simulink model "BallPlate"  (R2018b)
settings: Solver=VariableStepAuto  StartTime=0.0  StopTime=20  FixedStep=0.001  RelTol=1e-3
libraries: vrlib x6, aerolibanimutils x1
settings Model: Creator=enrico  LastModifiedBy=enrico

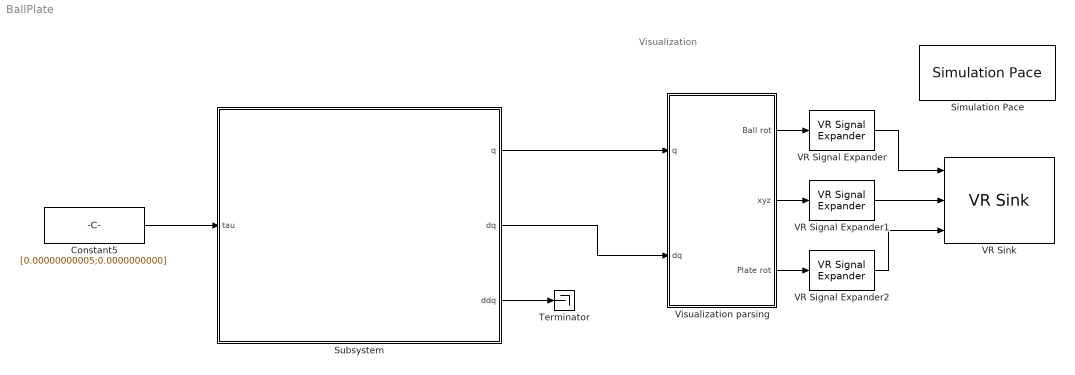
== system BallPlate ==
  note: Visualization
  Constant5 : Constant  Value=[0.00000000005;0.0000000000]
  Simulation Pace : aerolibanimutils/Simulation Pace  SimulationPace=1  SleepMode=Auto  OutputPaceError=off  SampleTime=1/30
  Subsystem : Subsystem
  Terminator : Terminator
  VR Signal Expander : vrlib/VR Signal Expander  outwidth=4  outidx=[1 2 3 4]
      settings: SourceProductName=Simulink 3D Animation  SourceProductBaseCode=VR
  VR Signal Expander1 : vrlib/VR Signal Expander  outwidth=3  outidx=[1 2 3]
      settings: SourceProductName=Simulink 3D Animation  SourceProductBaseCode=VR
  VR Signal Expander2 : vrlib/VR Signal Expander  outwidth=4  outidx=[1 2 3 4]
      settings: SourceProductName=Simulink 3D Animation  SourceProductBaseCode=VR
  VR Sink : vrlib/VR Sink  InstantiateOnLoad=on  SampleTime=-1  ViewEnable=on  RemoteChange=off  RemoteView=off  FieldsWritten=Ball.rotation.4.1.1.double#Ball.translation.3.1.1.double#Plate.rotation.4.1.1.double  WorldFileName=BallPlateVR.wrl  WorldDescription=Ball and plate  AutoView=on  VideoDimensions=[]  AllowVariableSize=off  mask(Virtual Reality Sink){}
      settings: SourceProductBaseCode=VR
  Visualization parsing : Subsystem
  wires:
  VR Signal Expander/1 -> VR Sink/1
  VR Signal Expander2/1 -> VR Sink/3
  Subsystem/1(q) -> Visualization parsing/1(q)
  Subsystem/2(dq) -> Visualization parsing/2(dq)
  Visualization parsing/1(Ball rot) -> VR Signal Expander/1
  VR Signal Expander1/1 -> VR Sink/2
  Subsystem/3(ddq) -> Terminator/1
  Visualization parsing/2(xyz) -> VR Signal Expander1/1
  Visualization parsing/3(Plate rot) -> VR Signal Expander2/1
  Constant5/1 -> Subsystem/1(tau)

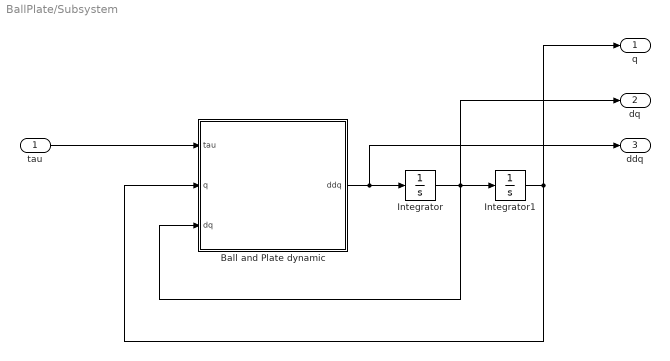
== system BallPlate/Subsystem ==
  tau : Inport
  Ball and Plate dynamic : MATLAB Function  TreatAsAtomicUnit=on
  Integrator : Integrator  InitialCondition=[0; 0; 0; 0]
  Integrator1 : Integrator  InitialCondition=[0; 0; 0; 0]
  q : Outport
  dq : Outport  Port=2
  ddq : Outport  Port=3
  wires:
  tau/1 -> Ball and Plate dynamic/1(tau)
  Integrator1/1 -> q/1, Ball and Plate dynamic/2(q)
  Integrator/1 -> Ball and Plate dynamic/3(dq), dq/1, Integrator1/1
  Ball and Plate dynamic/1(ddq) -> ddq/1, Integrator/1

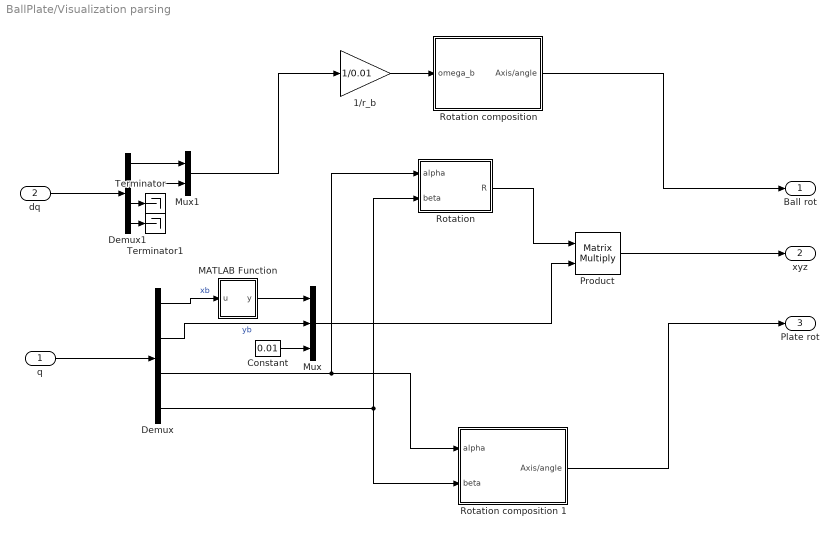
== system BallPlate/Visualization parsing ==
  q : Inport
  dq : Inport  Port=2
  1/r_b : Gain  Gain=1/0.01
  Constant : Constant  Value=0.01
  Demux : Demux
  Demux1 : Demux
  MATLAB Function : MATLAB Function  TreatAsAtomicUnit=on
  Mux : Mux  Inputs=3
  Mux1 : Mux  Inputs=2
  Product : Product  Multiplication=Matrix(*)
  Rotation : MATLAB Function  TreatAsAtomicUnit=on
  Rotation composition : Subsystem
  Rotation composition 1 : Subsystem
  Terminator : Terminator
  Terminator1 : Terminator
  Ball rot : Outport
  xyz : Outport  Port=2
  Plate rot : Outport  Port=3
  wires:
  Demux/2 -> Mux/2  "yb"
  1/r_b/1 -> Rotation composition/1(omega_b)
  Demux/3 -> Rotation/1(alpha), Rotation composition 1/1(alpha)
  dq/1 -> Demux1/1
  Mux1/1 -> 1/r_b/1
  Demux/1 -> MATLAB Function/1(u)  "xb"
  q/1 -> Demux/1
  Demux1/1 -> Mux1/1
  Demux1/4 -> Terminator1/1
  Rotation composition/1(Axis/angle) -> Ball rot/1
  Demux1/3 -> Terminator/1
  Demux/4 -> Rotation composition 1/2(beta), Rotation/2(beta)
  Rotation composition 1/1(Axis/angle) -> Plate rot/1
  Demux1/2 -> Mux1/2
  Constant/1 -> Mux/3
  Mux/1 -> Product/2
  Rotation/1(R) -> Product/1
  MATLAB Function/1(y) -> Mux/1
  Product/1 -> xyz/1

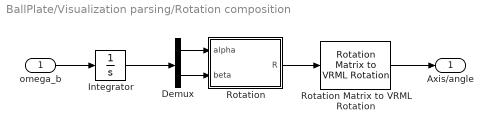
== system BallPlate/Visualization parsing/Rotation composition ==
  omega_b : Inport
  Demux : Demux  Outputs=2
  Integrator : Integrator  InitialCondition=[0; 0]
  Rotation : MATLAB Function  TreatAsAtomicUnit=on
  Rotation Matrix to VRML Rotation : vrlib/Utilities/Rotation Matrix to VRML Rotation  maxzero=1e-12
      settings: SourceProductName=Simulink 3D Animation  SourceProductBaseCode=VR
  Axis/angle : Outport
  wires:
  omega_b/1 -> Integrator/1
  Integrator/1 -> Demux/1
  Rotation Matrix to VRML Rotation/1 -> Axis/angle/1
  Rotation/1(R) -> Rotation Matrix to VRML Rotation/1
  Demux/1 -> Rotation/1(alpha)
  Demux/2 -> Rotation/2(beta)

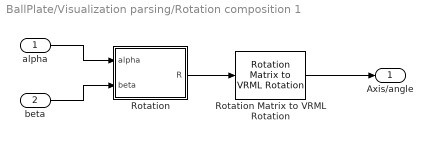
== system BallPlate/Visualization parsing/Rotation composition 1 ==
  alpha : Inport
  beta : Inport  Port=2
  Rotation : MATLAB Function  TreatAsAtomicUnit=on
  Rotation Matrix to VRML Rotation : vrlib/Utilities/Rotation Matrix to VRML Rotation  maxzero=1e-12
      settings: SourceProductName=Simulink 3D Animation  SourceProductBaseCode=VR
  Axis/angle : Outport
  wires:
  alpha/1 -> Rotation/1(alpha)
  Rotation Matrix to VRML Rotation/1 -> Axis/angle/1
  beta/1 -> Rotation/2(beta)
  Rotation/1(R) -> Rotation Matrix to VRML Rotation/1

== matlab function BallPlate/Visualization parsing/Rotation composition/Rotation ==
  data: alpha input; R output; beta input
function R = fcn(alpha, beta)

    alpha = -alpha;
    beta = -beta;
    Rx = [1 0 0; 0 cos(beta) -sin(beta); 0 sin(beta) cos(beta)];
    Ry = [cos(alpha) 0 sin(alpha); 0 1 0; -sin(alpha) 0 cos(alpha)];

R = Rx*Ry;

== matlab function BallPlate/Subsystem/Ball and Plate dynamic ==
  data: tau input; ddq output; q input; dq input
function ddq = InvDyn_BP(tau, q, dq)

if size(dq,2) == 3
    dq = dq';
end

tau1 = [0; 0; tau(1); tau(2)];

% B, C, G matrices
[B, C, G] = BCG_BP(q, dq);

% Inverse dynamic
ddq = B\(tau1 - C*dq - G); 

end

== matlab function BallPlate/Visualization parsing/Rotation composition 1/Rotation ==
  data: alpha input; R output; beta input
function R = fcn(alpha, beta)
    
    Rx = [1 0 0; 0 cos(beta) -sin(beta); 0 sin(beta) cos(beta)];
    Ry = [cos(alpha) 0 sin(alpha); 0 1 0; -sin(alpha) 0 cos(alpha)];

R = Rx*Ry;

== matlab function BallPlate/Visualization parsing/Rotation ==
  data: alpha input; R output; beta input
function R = fcn(alpha, beta)

    Rx = [1 0 0; 0 cos(beta) -sin(beta); 0 sin(beta) cos(beta)];
    Ry = [cos(alpha) 0 sin(alpha); 0 1 0; -sin(alpha) 0 cos(alpha)];

R = Rx*Ry;

== matlab function BallPlate/Visualization parsing/MATLAB Function ==
  data: u input; y output
function y = fcn(u)

y = -u;
